simulink model "exercise_04_10_sim_fbk"  (R2020b)
settings: Solver=ode4  StartTime=0.0  StopTime=10  FixedStep=0.001  RelTol=1e-3
undefined symbols (not defined in the file): dc, rc
settings Model: Creator=kawata  LastModifiedBy=kawata
settings DataIOCC: ReturnWorkspaceOutputs=off

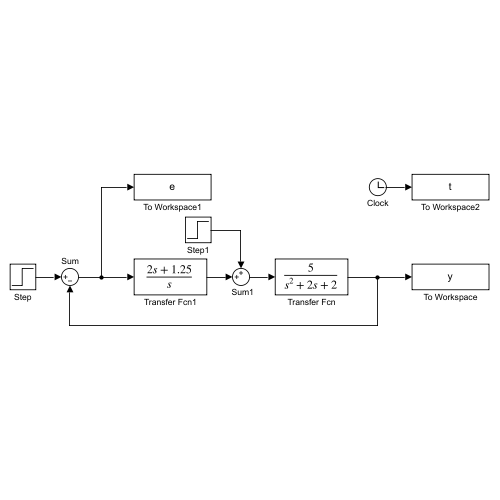
[thumbnail: Simulink's stored preview of the top-level diagram]
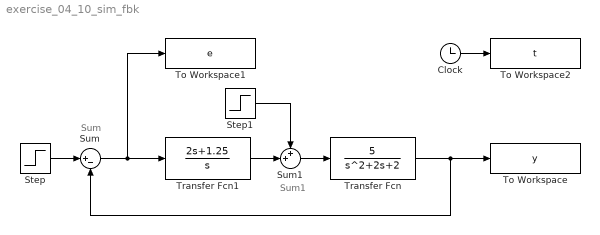
== system exercise_04_10_sim_fbk ==
  note: Sum
  note: Sum1
  Clock : Clock
  Step : Step  Time=0  After=rc  SampleTime=0
  Step1 : Step  Time=0  After=dc  SampleTime=0
  Sum : Sum  Inputs=|+-
  Sum1 : Sum  Inputs=++|
  To Workspace : ToWorkspace  VariableName=y  SampleTime=-1
  To Workspace1 : ToWorkspace  VariableName=e  SampleTime=-1
  To Workspace2 : ToWorkspace  VariableName=t  SampleTime=-1
  Transfer Fcn : TransferFcn  Numerator=[5]  Denominator=[1 2 2]
  Transfer Fcn1 : TransferFcn  Numerator=[2 1.25]  Denominator=[1 0]
  wires:
  Step/1 -> Sum/1
  Sum/1 -> Transfer Fcn1/1, To Workspace1/1
  Transfer Fcn1/1 -> Sum1/2
  Step1/1 -> Sum1/1
  Sum1/1 -> Transfer Fcn/1
  Transfer Fcn/1 -> To Workspace/1, Sum/2
  Clock/1 -> To Workspace2/1
